simulink model "gm_FOC"  (R2020a)
settings: Solver=FixedStepAuto  StartTime=0.0  StopTime=10.0  RelTol=1e-3
libraries: hdlmdlgenlib x12
(part 2 of 2)

== system gm_FOC/dq2abc/Inverse Park Transform/b/subtract1 ==
  In1 : Inport
  In2 : Inport  Port=2
  subtract1 : Sum  Inputs=+-  OutDataTypeStr=single  SampleTime=10000
  Out1 : Outport
  wires:
  In1/1 -> subtract1/1
  In2/1 -> subtract1/2
  subtract1/1 -> Out1/1

== system gm_FOC/dq2abc/Inverse Park Transform/c/adder ==
  In1 : Inport
  In2 : Inport  Port=2
  adder : Sum  OutDataTypeStr=single  SampleTime=10000
  Out1 : Outport
  wires:
  In1/1 -> adder/1
  In2/1 -> adder/2
  adder/1 -> Out1/1

== system gm_FOC/dq2abc/Inverse Park Transform/c/adder1 ==
  In1 : Inport
  In2 : Inport  Port=2
  adder1 : Sum  OutDataTypeStr=single  SampleTime=10000
  Out1 : Outport
  wires:
  In1/1 -> adder1/1
  In2/1 -> adder1/2
  adder1/1 -> Out1/1

== system gm_FOC/dq2abc/Inverse Park Transform/c/adder2 ==
  In1 : Inport
  In2 : Inport  Port=2
  adder2 : Sum  OutDataTypeStr=single  SampleTime=10000
  Out1 : Outport
  wires:
  In1/1 -> adder2/1
  In2/1 -> adder2/2
  adder2/1 -> Out1/1

== system gm_FOC/dq2abc/Inverse Park Transform/c/adder3 ==
  In1 : Inport
  In2 : Inport  Port=2
  adder3 : Sum  OutDataTypeStr=single  SampleTime=10000
  Out1 : Outport
  wires:
  In1/1 -> adder3/1
  In2/1 -> adder3/2
  adder3/1 -> Out1/1

== system gm_FOC/dq2abc/Inverse Park Transform/c/adder4 ==
  In1 : Inport
  In2 : Inport  Port=2
  adder4 : Sum  OutDataTypeStr=single  SampleTime=10000
  Out1 : Outport
  wires:
  In1/1 -> adder4/1
  In2/1 -> adder4/2
  adder4/1 -> Out1/1

== system gm_FOC/dq2abc/Inverse Park Transform/c/adder5 ==
  In1 : Inport
  In2 : Inport  Port=2
  adder5 : Sum  OutDataTypeStr=single  SampleTime=10000
  Out1 : Outport
  wires:
  In1/1 -> adder5/1
  In2/1 -> adder5/2
  adder5/1 -> Out1/1

== system gm_FOC/dq2abc/Inverse Park Transform/c/cos ==
  In1 : Inport
  cos : Trigonometry  Operator=cos  SampleTime=10000
  Out1 : Outport
  wires:
  In1/1 -> cos/1
  cos/1 -> Out1/1

== system gm_FOC/dq2abc/Inverse Park Transform/c/multiplier ==
  In1 : Inport
  In2 : Inport  Port=2
  multiplier : Product  Inputs=**  OutDataTypeStr=single  SampleTime=10000
  Out1 : Outport
  wires:
  In1/1 -> multiplier/1
  In2/1 -> multiplier/2
  multiplier/1 -> Out1/1

== system gm_FOC/dq2abc/Inverse Park Transform/c/multiplier1 ==
  In1 : Inport
  In2 : Inport  Port=2
  multiplier1 : Product  Inputs=**  OutDataTypeStr=single  SampleTime=10000
  Out1 : Outport
  wires:
  In1/1 -> multiplier1/1
  In2/1 -> multiplier1/2
  multiplier1/1 -> Out1/1

== system gm_FOC/dq2abc/Inverse Park Transform/c/sin ==
  In1 : Inport
  sin : Trigonometry  SampleTime=10000
  Out1 : Outport
  wires:
  In1/1 -> sin/1
  sin/1 -> Out1/1
